simulink model "rosdemo"  (Simulink 7.1)
settings: Solver=ode5  StartTime=0.0  StopTime=20  FixedStep=1e-3  RelTol=1e-3
undefined symbols (not defined in the file): sigbuilder_block
libraries: rtairos x12, simulink x3, simulink_extras x1
Description:
  | RTAI-ROS demonstration model
settings Model: Creator=rhopfer  LastModifiedBy=rho
settings HardwareCC: TargetBitPerLong=64  TargetEndianess=LittleEndian  TargetWordSize=64  TargetHWDeviceType=MATLAB Host  ProdEqTarget=off
settings RTWCC: SystemTargetFile=rtairos.tlc  GenCodeOnly=on  TemplateMakefile=rtairos.tmf  Description=Linux RTAI Real-Time Target with ROS  TLCAssert=on  ProcessScript=rtairos_make_rtw_hook
settings STFCustomTargetCC: ModelReferenceCompliant=off  MatFileLogging=on  SystemTargetFile=rtairos.tlc
settings CustomProperty: DataType=string  Value=demo
settings EnumStrPairs: String=no

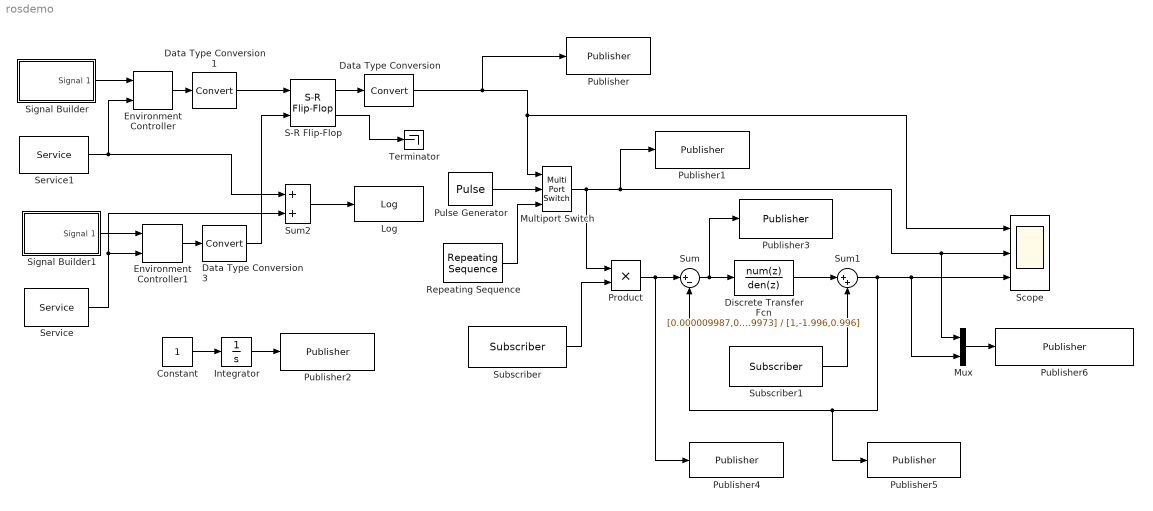
== system rosdemo ==
  Constant : Constant  OutDataType=sfix(16)  OutScaling=2^0
  Data Type Conversion : DataTypeConversion  OutDataType=sfix(16)  OutScaling=2^0
  Data Type Conversion1 : DataTypeConversion  OutDataType=sfix(16)  OutScaling=2^0
  Data Type Conversion3 : DataTypeConversion  OutDataType=sfix(16)  OutScaling=2^0
  Discrete Transfer Fcn : DiscreteTransferFcn  Numerator=[0.000009987,0.000009973]  Denominator=[1,-1.996,0.996]  SampleTime=1e-3
  Environment Controller : simulink/Signal Routing/Environment Controller  SystemSampleTime=-1
  Environment Controller1 : simulink/Signal Routing/Environment Controller  SystemSampleTime=-1
  Integrator : Integrator
  Log : rtairos/ROS/Log  level=info  msg=Source signal changed  dataport=off
  Multiport Switch : MultiPortSwitch  Inputs=2  zeroidx=on  OutDataType=sfix(16)  OutScaling=2^0
  Mux : Mux  Inputs=2
  Product : Product  OutDataType=sfix(16)  OutScaling=2^0  RndMeth=Zero
  Publisher : rtairos/ROS/Publisher  msgtype=std_msgs/Int32  topic=signal  sampleTime=-1
  Publisher1 : rtairos/ROS/Publisher  msgtype=std_msgs/Float64  topic=u  sampleTime=-1
  Publisher2 : rtairos/ROS/Publisher  msgtype=std_msgs/Time  topic=time  sampleTime=-1
  Publisher3 : rtairos/ROS/Publisher  msgtype=std_msgs/Float64  topic=e  sampleTime=-1
  Publisher4 : rtairos/ROS/Publisher  msgtype=std_msgs/Float64  topic=r  sampleTime=-1
  Publisher5 : rtairos/ROS/Publisher  msgtype=std_msgs/Float64  topic=y  sampleTime=-1
  Publisher6 : rtairos/ROS/Publisher  msgtype=std_msgs/Float64MultiArray  topic=uy  sampleTime=-1
  Pulse Generator : DiscretePulseGenerator  Period=10000  PulseWidth=5000  SampleTime=1e-3
  Repeating Sequence : simulink/Sources/Repeating Sequence  SystemSampleTime=-1  rep_seq_t=[0 2 4 6]  rep_seq_y=[0 2 2 0]
  S-R Flip-Flop : simulink_extras/Flip Flops/S-R Flip-Flop  SystemSampleTime=-1  initial_condition=0
  Scope : Scope  NumInputPorts=3
      settings: YMin=-5~-5~-5  YMax=5~5~5
  Service : rtairos/ROS/Service  srv=rectangle  sampleTime=-1
  Service1 : rtairos/ROS/Service  srv=trapezoid  sampleTime=-1
  Signal Builder : Subsystem  Tag=STV Subsys  LoadFcn=sigbuilder_block('load');  StartFcn=sigbuilder_block('start');  StopFcn=sigbuilder_block('stop');  ClipboardFcn=sigbuilder_block('clipboard');  mask(Sigbuilder block){}
      mask help: Sigbuilder GUI
      mask init:
      | if ~strcmp(get_param(bdroot(gcbh),'SimulationStatus'),'stopped') tuvar = sigbuilder_block('maskInit'); end
      settings: CopyFcn=sigbuilder_block('copy');  DeleteFcn=sigbuilder_block('delete');  ModelCloseFcn=sigbuilder_block('modelClose');  PreSaveFcn=sigbuilder_block('preSave');  NameChangeFcn=sigbuilder_block('namechange');  OpenFcn=sigbuilder_block('open',[437.6 199.2 550.4 400 ]);  CloseFcn=sigbuilder_block('close');
      mask Display: plot(0,0,100,100,[10,10,40,40,10],[80,20,20,80,80],[40,10],[50,50], [40,27,10],[65,72,56],[40,25,25,10],[28,28,43,43]);
  Signal Builder1 : Subsystem  Tag=STV Subsys  LoadFcn=sigbuilder_block('load');  StartFcn=sigbuilder_block('start');  StopFcn=sigbuilder_block('stop');  ClipboardFcn=sigbuilder_block('clipboard');  mask(Sigbuilder block){}
      mask help: Sigbuilder GUI
      mask init:
      | if ~strcmp(get_param(bdroot(gcbh),'SimulationStatus'),'stopped') tuvar = sigbuilder_block('maskInit'); end
      settings: CopyFcn=sigbuilder_block('copy');  DeleteFcn=sigbuilder_block('delete');  ModelCloseFcn=sigbuilder_block('modelClose');  PreSaveFcn=sigbuilder_block('preSave');  NameChangeFcn=sigbuilder_block('namechange');  OpenFcn=sigbuilder_block('open',[437.6 199.2 550.4 400 ]);  CloseFcn=sigbuilder_block('close');
      mask Display: plot(0,0,100,100,[10,10,40,40,10],[80,20,20,80,80],[40,10],[50,50], [40,27,10],[65,72,56],[40,25,25,10],[28,28,43,43]);
  Subscriber : rtairos/ROS/Subscriber  msgtype=std_msgs/Float64  topic=v  initval=1  sampleTime=-1  reset=off
  Subscriber1 : rtairos/ROS/Subscriber  msgtype=std_msgs/Float64  topic=d  initval=0  sampleTime=-1  reset=off
  Sum : Sum  Inputs=|+-  OutDataType=sfix(16)  OutScaling=2^0  SaturateOnIntegerOverflow=on
  Sum1 : Sum  Inputs=|++  OutDataType=sfix(16)  OutScaling=2^0  SaturateOnIntegerOverflow=on
  Sum2 : Sum  OutDataType=sfix(16)  OutScaling=2^0  SaturateOnIntegerOverflow=on
  Terminator : Terminator
  wires:
  Product/1 -> Sum/1, Publisher4/1
  Sum/1 -> Discrete Transfer Fcn/1, Publisher3/1
  Subscriber/1 -> Product/2
  Pulse Generator/1 -> Multiport Switch/2
  Repeating Sequence/1 -> Multiport Switch/3
  Multiport Switch/1 -> Product/1, Publisher1/1, Mux/1, Scope/2
  S-R Flip-Flop/1 -> Data Type Conversion/1
  Data Type Conversion/1 -> Multiport Switch/1, Scope/1, Publisher/1
  Data Type Conversion1/1 -> S-R Flip-Flop/1
  S-R Flip-Flop/2 -> Terminator/1
  Signal Builder/1(Signal 1) -> Environment Controller/1
  Signal Builder1/1(Signal 1) -> Environment Controller1/1
  Environment Controller1/1 -> Data Type Conversion3/1
  Service1/1 -> Environment Controller/2, Sum2/1
  Service/1 -> Environment Controller1/2, Sum2/2
  Data Type Conversion3/1 -> S-R Flip-Flop/2
  Discrete Transfer Fcn/1 -> Sum1/1
  Subscriber1/1 -> Sum1/2
  Sum1/1 -> Sum/2, Publisher5/1, Mux/2, Scope/3
  Mux/1 -> Publisher6/1
  Environment Controller/1 -> Data Type Conversion1/1
  Sum2/1 -> Log/1
  Constant/1 -> Integrator/1
  Integrator/1 -> Publisher2/1

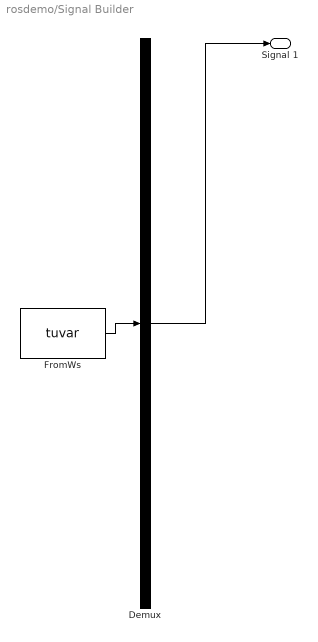
== system rosdemo/Signal Builder ==
  Demux : Demux  Tag=STV Demux  Outputs=1
  FromWs : FromWorkspace  Tag=STV FromWs  VariableName=tuvar  SampleTime=0  SigBuilderData=DataTag0  VnvData=DataTag1
      SigBuilderData=|
      | common.afterFinalStr = 'Extrapolate'
      | common.sampleTime = 0
      | dataSet.timeRange = [0 10]
      | dataSet.name = 'Group 1'
      | sbobj.Groups{1}.Signals{1}.XData = [0 8 8 8.14 8.14 10]
      | sbobj.Groups{1}.Signals{1}.YData = [0 0 1 1 0 0]
  Signal 1 : Outport  Tag=STV Outport  OutDataType=sfix(16)  OutScaling=2^0
  wires:
  Demux/1 -> Signal 1/1
  FromWs/1 -> Demux/1

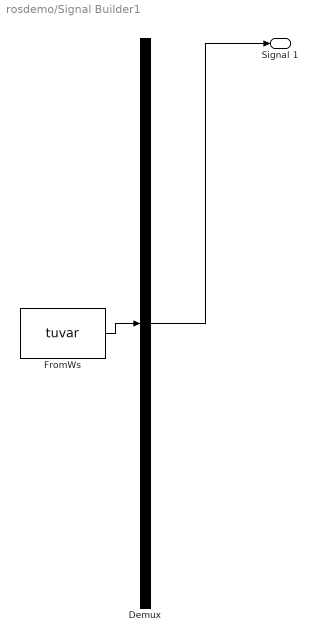
== system rosdemo/Signal Builder1 ==
  Demux : Demux  Tag=STV Demux  Outputs=1
  FromWs : FromWorkspace  Tag=STV FromWs  VariableName=tuvar  SampleTime=0  SigBuilderData=DataTag2  VnvData=DataTag3
      SigBuilderData=|
      | common.afterFinalStr = 'Extrapolate'
      | common.sampleTime = 0
      | dataSet.timeRange = [0 20]
      | dataSet.name = 'Group 1'
      | sbobj.Groups{1}.Signals{1}.XData = [0 14.05 14.05 14.3 14.3 20]
      | sbobj.Groups{1}.Signals{1}.YData = [0 0 1 1 0 0]
  Signal 1 : Outport  Tag=STV Outport  OutDataType=sfix(16)  OutScaling=2^0
  wires:
  FromWs/1 -> Demux/1
  Demux/1 -> Signal 1/1
